simulink model "LE3_3"  (R2018a)
settings: Solver=ode4  StartTime=0.0  StopTime=10.0  FixedStep=0.01  RelTol=1e-3
libraries: simulink x1
settings Model: Creator=Kenneth  LastModifiedBy=Kenneth

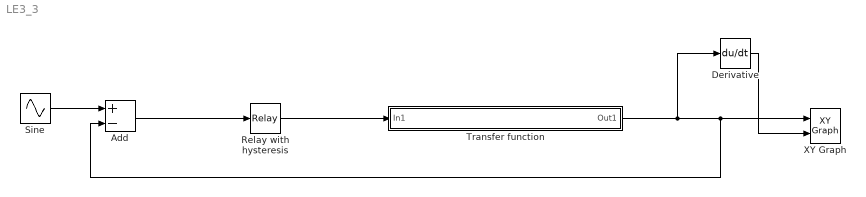
== system LE3_3 ==
  Add : Sum  Inputs=+-
  Derivative : Derivative
  Relay with hysteresis : Relay  OnSwitchValue=1  OffSwitchValue=-1  OnOutputValue=2  OffOutputValue=-2
  Sine : Sin  Frequency=1/(2*pi)  SampleTime=0
  Transfer function : Subsystem
  XY Graph : simulink/Sinks/XY Graph  xmin=-1  xmax=1  ymin=-1  ymax=1  st=-1
  wires:
  Derivative/1 -> XY Graph/2
  Sine/1 -> Add/1
  Add/1 -> Relay with hysteresis/1
  Transfer function/1(Out1) -> Add/2, XY Graph/1, Derivative/1
  Relay with hysteresis/1 -> Transfer function/1(In1)

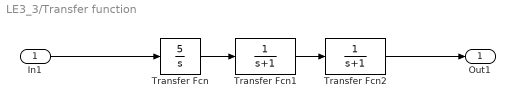
== system LE3_3/Transfer function ==
  In1 : Inport
  Transfer Fcn : TransferFcn  Numerator=[5]  Denominator=[1 0]
  Transfer Fcn1 : TransferFcn  Denominator=[1 1]
  Transfer Fcn2 : TransferFcn  Denominator=[1 1]
  Out1 : Outport
  wires:
  Transfer Fcn1/1 -> Transfer Fcn2/1
  Transfer Fcn/1 -> Transfer Fcn1/1
  Transfer Fcn2/1 -> Out1/1
  In1/1 -> Transfer Fcn/1
